simulink model "active_stereo_ibvs"  (R2025b)
settings: Solver=FixedStepDiscrete  StartTime=0.0  StopTime=Tstop  FixedStep=Ts  RelTol=1e-3
values from neighbouring files (symbols this model uses):
  Ts = cfg.Ts;'    [build_arm_stereo_ibvs_ekf_v1.m]
undefined symbols (not defined in the file or in its folder): adaptEnable, cam, dhatn0, DiscIntNeverNeededParam, experimentMode, featureScale, feedforwardEnable, gammaRho, lambda, mu, q0, qmax, qmin, rateScale, rho0, rhomax, rhomin, sd, sdDot, sigmaRho, target0, trajParam
settings Model: Creator=ASUS  LastModifiedBy=ASUS

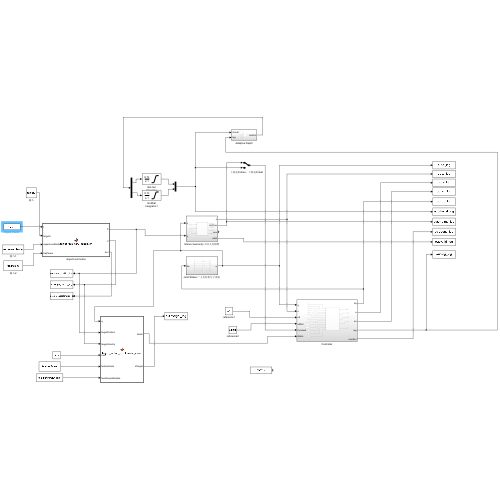
[thumbnail: Simulink's stored preview of the top-level diagram]
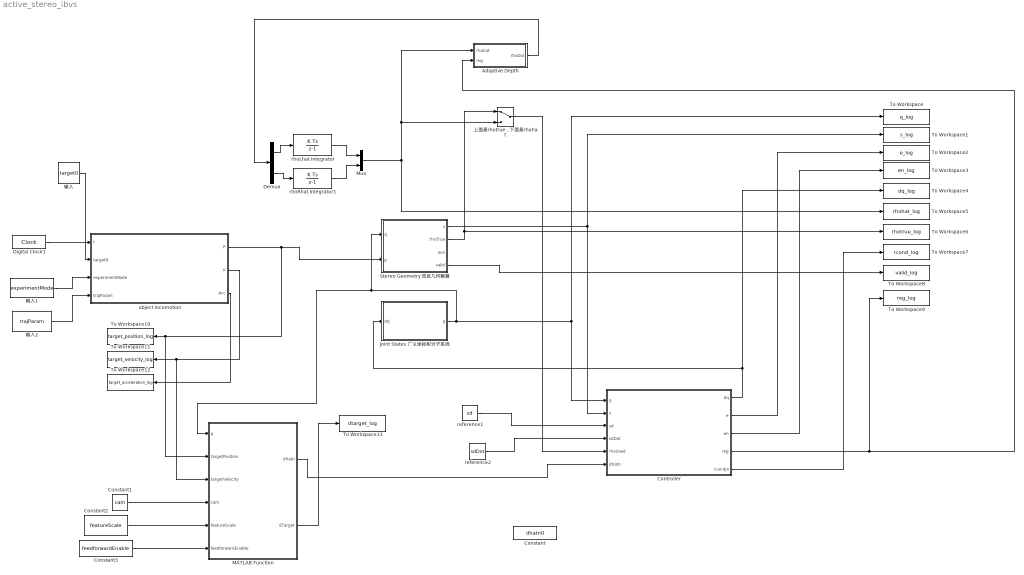
== system active_stereo_ibvs ==
  Adaptive Depth : Subsystem
  Constant : Constant  Value=dhatn0
  Constant1 : Constant  Value=cam
  Constant2 : Constant  Value=featureScale
  Constant3 : Constant  Value=feedforwardEnable
  Controller : Subsystem
  Demux : Demux  Outputs=2
  Digital Clock1 : DigitalClock  SampleTime=Ts
  Joint States 广义坐标积分子系统 : Subsystem
  MATLAB Function : MATLAB Function  TreatAsAtomicUnit=on
  Mux : Mux  Inputs=2
  Stereo Geometry 双目几何解算 : Subsystem
  To Workspace : ToWorkspace  VariableName=q_log  SaveFormat=Timeseries  SampleTime=-1
  To Workspace1 : ToWorkspace  VariableName=s_log  SaveFormat=Timeseries  SampleTime=-1
  To Workspace10 : ToWorkspace  VariableName=target_position_log  SaveFormat=Timeseries  SampleTime=-1
  To Workspace11 : ToWorkspace  VariableName=target_velocity_log  SaveFormat=Timeseries  SampleTime=-1
  To Workspace12 : ToWorkspace  VariableName=target_acceleration_log  SaveFormat=Timeseries  SampleTime=-1
  To Workspace13 : ToWorkspace  VariableName=dtarget_log  SaveFormat=Timeseries  SampleTime=-1
  To Workspace2 : ToWorkspace  VariableName=e_log  SaveFormat=Timeseries  SampleTime=-1
  To Workspace3 : ToWorkspace  VariableName=en_log  SaveFormat=Timeseries  SampleTime=-1
  To Workspace4 : ToWorkspace  VariableName=dq_log  SaveFormat=Timeseries  SampleTime=-1
  To Workspace5 : ToWorkspace  VariableName=rhohat_log  SaveFormat=Timeseries  SampleTime=-1
  To Workspace6 : ToWorkspace  VariableName=rhotrue_log  SaveFormat=Timeseries  SampleTime=-1
  To Workspace7 : ToWorkspace  VariableName=rcond_log  SaveFormat=Timeseries  SampleTime=-1
  To Workspace8 : ToWorkspace  VariableName=valid_log  SaveFormat=Timeseries  SampleTime=-1
  To Workspace9 : ToWorkspace  VariableName=reg_log  SaveFormat=Timeseries  SampleTime=-1
  object locomotion : MATLAB Function  TreatAsAtomicUnit=on
  reference1 : Constant  Value=sd
  reference2 : Constant  Value=sdDot
  rhoLhat Integrator : DiscreteIntegrator  InitialCondition=rho0(1)  SampleTime=Ts  LimitOutput=on  UpperSaturationLimit=rhomax(1)  LowerSaturationLimit=rhomin(1)  ICPrevOutput=DiscIntNeverNeededParam  ICPrevScaledInput=DiscIntNeverNeededParam
  rhoRhat Integrator1 : DiscreteIntegrator  InitialCondition=rho0(2)  SampleTime=Ts  LimitOutput=on  UpperSaturationLimit=rhomax(2)  LowerSaturationLimit=rhomin(2)  ICPrevOutput=DiscIntNeverNeededParam  ICPrevScaledInput=DiscIntNeverNeededParam
  上面是rhotrue，下面是rhohat : ManualSwitch
  输入 : Constant  Value=target0
  输入1 : Constant  Value=experimentMode
  输入2 : Constant  Value=trajParam
  wires:
  rhoLhat Integrator/1 -> Mux/1
  rhoRhat Integrator1/1 -> Mux/2
  Mux/1 -> Adaptive Depth/1(rhohat), 上面是rhotrue，下面是rhohat/2, To Workspace5/1
  Controller/1(dq) -> To Workspace4/1, Joint States 广义坐标积分子系统/1(dq)
  Stereo Geometry 双目几何解算/2(rhoTrue) -> To Workspace6/1, 上面是rhotrue，下面是rhohat/1
  上面是rhotrue，下面是rhohat/1 -> Controller/5(rhoUsed)
  Joint States 广义坐标积分子系统/1(q) -> MATLAB Function/1(q), Stereo Geometry 双目几何解算/1(q), Controller/1(q), To Workspace/1
  Stereo Geometry 双目几何解算/1(s) -> Controller/2(s), To Workspace1/1
  Controller/2(e) -> To Workspace2/1
  Controller/3(en) -> To Workspace3/1
  Controller/5(rcondJn) -> To Workspace7/1
  Stereo Geometry 双目几何解算/4(valid) -> To Workspace8/1
  Demux/1 -> rhoLhat Integrator/1
  Demux/2 -> rhoRhat Integrator1/1
  Adaptive Depth/1(rhoDot) -> Demux/1
  Controller/4(reg) -> To Workspace9/1, Adaptive Depth/2(reg)
  reference1/1 -> Controller/3(sd)
  reference2/1 -> Controller/4(sdDot)
  Digital Clock1/1 -> object locomotion/1(t)
  输入/1 -> object locomotion/2(target0)
  输入1/1 -> object locomotion/3(experimentMode)
  输入2/1 -> object locomotion/4(trajParam)
  object locomotion/1(P) -> MATLAB Function/2(targetPosition), To Workspace10/1, Stereo Geometry 双目几何解算/2(p)
  object locomotion/2(V) -> MATLAB Function/3(targetVelocity), To Workspace11/1
  object locomotion/3(Acc) -> To Workspace12/1
  Constant1/1 -> MATLAB Function/4(cam)
  Constant2/1 -> MATLAB Function/5(featureScale)
  Constant3/1 -> MATLAB Function/6(feedforwardEnable)
  MATLAB Function/2(dTarget) -> To Workspace13/1
  MATLAB Function/1(dhatn) -> Controller/6(dhatn)

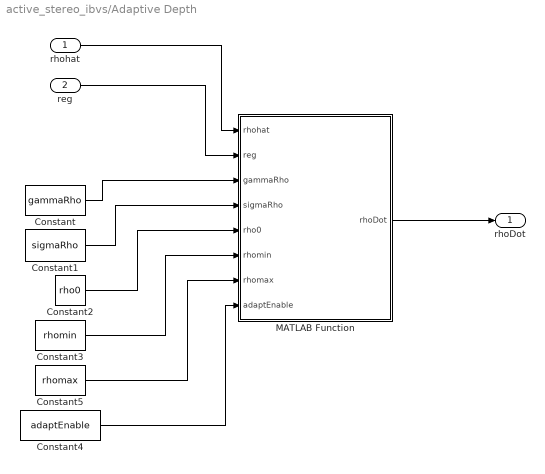
== system active_stereo_ibvs/Adaptive Depth ==
  rhohat : Inport
  reg : Inport  Port=2
  Constant : Constant  Value=gammaRho
  Constant1 : Constant  Value=sigmaRho
  Constant2 : Constant  Value=rho0
  Constant3 : Constant  Value=rhomin
  Constant4 : Constant  Value=adaptEnable
  Constant5 : Constant  Value=rhomax
  MATLAB Function : MATLAB Function  TreatAsAtomicUnit=on
  rhoDot : Outport
  wires:
  rhohat/1 -> MATLAB Function/1(rhohat)
  reg/1 -> MATLAB Function/2(reg)
  MATLAB Function/1(rhoDot) -> rhoDot/1
  Constant/1 -> MATLAB Function/3(gammaRho)
  Constant1/1 -> MATLAB Function/4(sigmaRho)
  Constant2/1 -> MATLAB Function/5(rho0)
  Constant3/1 -> MATLAB Function/6(rhomin)
  Constant5/1 -> MATLAB Function/7(rhomax)
  Constant4/1 -> MATLAB Function/8(adaptEnable)

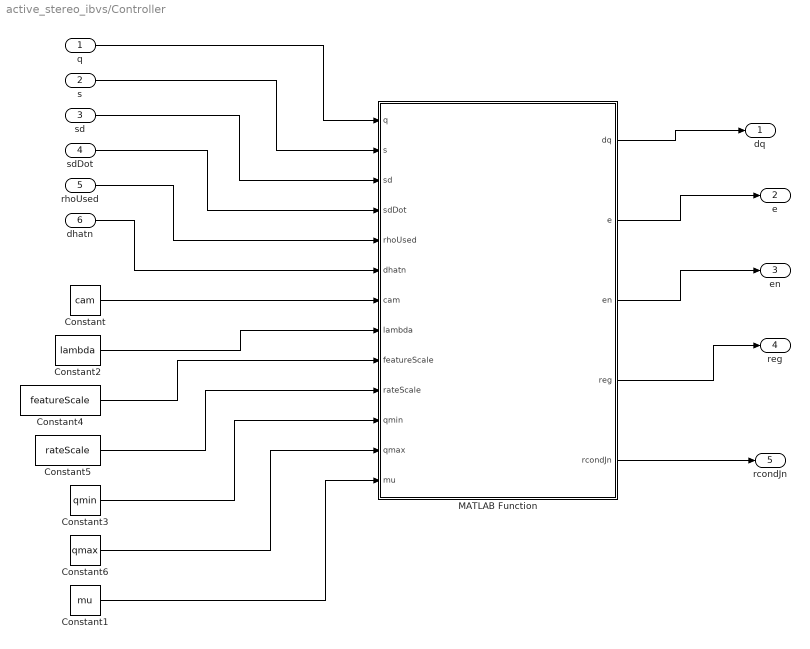
== system active_stereo_ibvs/Controller ==
  q : Inport
  s : Inport  Port=2
  sd : Inport  Port=3
  sdDot : Inport  Port=4
  rhoUsed : Inport  Port=5
  dhatn : Inport  Port=6
  Constant : Constant  Value=cam
  Constant1 : Constant  Value=mu
  Constant2 : Constant  Value=lambda
  Constant3 : Constant  Value=qmin  VectorParams1D=off
  Constant4 : Constant  Value=featureScale
  Constant5 : Constant  Value=rateScale
  Constant6 : Constant  Value=qmax
  MATLAB Function : MATLAB Function  TreatAsAtomicUnit=on
  dq : Outport
  e : Outport  Port=2
  en : Outport  Port=3
  reg : Outport  Port=4
  rcondJn : Outport  Port=5
  wires:
  q/1 -> MATLAB Function/1(q)
  s/1 -> MATLAB Function/2(s)
  sd/1 -> MATLAB Function/3(sd)
  sdDot/1 -> MATLAB Function/4(sdDot)
  rhoUsed/1 -> MATLAB Function/5(rhoUsed)
  dhatn/1 -> MATLAB Function/6(dhatn)
  Constant/1 -> MATLAB Function/7(cam)
  Constant2/1 -> MATLAB Function/8(lambda)
  Constant4/1 -> MATLAB Function/9(featureScale)
  Constant5/1 -> MATLAB Function/10(rateScale)
  Constant3/1 -> MATLAB Function/11(qmin)
  Constant6/1 -> MATLAB Function/12(qmax)
  Constant1/1 -> MATLAB Function/13(mu)
  MATLAB Function/1(dq) -> dq/1
  MATLAB Function/2(e) -> e/1
  MATLAB Function/3(en) -> en/1
  MATLAB Function/4(reg) -> reg/1
  MATLAB Function/5(rcondJn) -> rcondJn/1

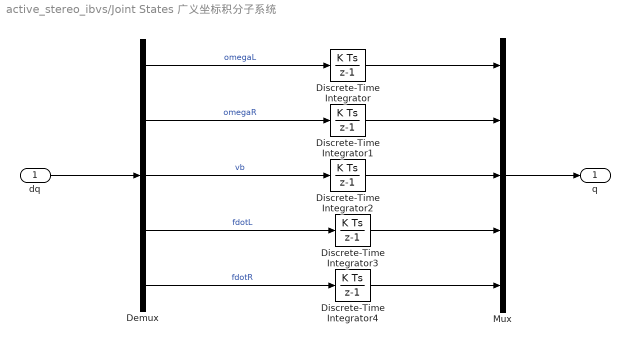
== system active_stereo_ibvs/Joint States 广义坐标积分子系统 ==
  dq : Inport
  Demux : Demux  Outputs=5
  Discrete-Time Integrator : DiscreteIntegrator  InitialCondition=q0(1)  SampleTime=Ts  LimitOutput=on  UpperSaturationLimit=qmax(1)  LowerSaturationLimit=qmin(1)  ICPrevOutput=DiscIntNeverNeededParam  ICPrevScaledInput=DiscIntNeverNeededParam
  Discrete-Time Integrator1 : DiscreteIntegrator  InitialCondition=q0(2)  SampleTime=Ts  LimitOutput=on  UpperSaturationLimit=qmax(2)  LowerSaturationLimit=qmin(2)  ICPrevOutput=DiscIntNeverNeededParam  ICPrevScaledInput=DiscIntNeverNeededParam
  Discrete-Time Integrator2 : DiscreteIntegrator  InitialCondition=q0(3)  SampleTime=Ts  LimitOutput=on  UpperSaturationLimit=qmax(3)  LowerSaturationLimit=qmin(3)  ICPrevOutput=DiscIntNeverNeededParam  ICPrevScaledInput=DiscIntNeverNeededParam
  Discrete-Time Integrator3 : DiscreteIntegrator  InitialCondition=q0(4)  SampleTime=Ts  LimitOutput=on  UpperSaturationLimit=qmax(4)  LowerSaturationLimit=qmin(4)  ICPrevOutput=DiscIntNeverNeededParam  ICPrevScaledInput=DiscIntNeverNeededParam
  Discrete-Time Integrator4 : DiscreteIntegrator  InitialCondition=q0(5)  SampleTime=Ts  LimitOutput=on  UpperSaturationLimit=qmax(5)  LowerSaturationLimit=qmin(5)  ICPrevOutput=DiscIntNeverNeededParam  ICPrevScaledInput=DiscIntNeverNeededParam
  Mux : Mux  Inputs=5
  q : Outport
  wires:
  Demux/4 -> Discrete-Time Integrator3/1  "fdotL"
  Demux/3 -> Discrete-Time Integrator2/1  "vb"
  Demux/5 -> Discrete-Time Integrator4/1  "fdotR"
  Discrete-Time Integrator4/1 -> Mux/5
  Discrete-Time Integrator1/1 -> Mux/2
  Discrete-Time Integrator/1 -> Mux/1
  Discrete-Time Integrator2/1 -> Mux/3
  Discrete-Time Integrator3/1 -> Mux/4
  Demux/2 -> Discrete-Time Integrator1/1  "omegaR"
  Demux/1 -> Discrete-Time Integrator/1  "omegaL"
  dq/1 -> Demux/1
  Mux/1 -> q/1

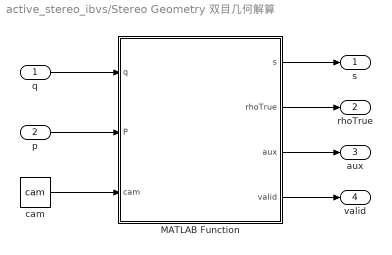
== system active_stereo_ibvs/Stereo Geometry 双目几何解算 ==
  q : Inport
  p : Inport  Port=2
  MATLAB Function : MATLAB Function  TreatAsAtomicUnit=on
  cam : Constant  Value=cam
  s : Outport
  rhoTrue : Outport  Port=2
  aux : Outport  Port=3
  valid : Outport  Port=4
  wires:
  q/1 -> MATLAB Function/1(q)
  p/1 -> MATLAB Function/2(P)
  cam/1 -> MATLAB Function/3(cam)
  MATLAB Function/1(s) -> s/1
  MATLAB Function/2(rhoTrue) -> rhoTrue/1
  MATLAB Function/3(aux) -> aux/1
  MATLAB Function/4(valid) -> valid/1

== matlab function active_stereo_ibvs/Controller/MATLAB Function ==
  data: q input; dq output size=[5 1]; s input; sd input; sdDot input; rhoUsed input; dhatn input; cam input; lambda input; featureScale input; rateScale input; qmin input; qmax input; mu input; e output; en output; reg output; rcondJn output
function [dq, e, en, reg, rcondJn] = controller5( ...
    q, s, sd, sdDot, rhoUsed, dhatn, ...
    cam, lambda, featureScale, rateScale, qmin, qmax, mu)
%#codegen
%
% q  = [alphaL; alphaR; b; fL; fR]
% s  = [uL; aL; uR; aR; b]
% dq = [omegaL; omegaR; vb; fdotL; fdotR]

%% 固定输出尺寸
dq = zeros(5,1);
e = zeros(5,1);
en = zeros(5,1);
reg = zeros(2,1);
rcondJn = 0.0;

%% 固定中间变量尺寸
W = zeros(5,5);
Du = zeros(5,5);
Jhat = zeros(5,5);
Jn = zeros(5,5);
G = zeros(5,5);
rhs = zeros(5,1);
z = zeros(5,1);

JL = zeros(5,5);
JR = zeros(5,5);
phiL = zeros(5,1);
phiR = zeros(5,1);

%% 读取状态
alphaL = q(1);
alphaR = q(2);

fL = q(4);
fR = q(5);

uL = s(1);
aL = s(2);
uR = s(3);
aR = s(4);

cxL = cam(1);
cxR = cam(2);

rhoL = rhoUsed(1);
rhoR = rhoUsed(2);

sigmaL = -1.0;
sigmaR =  1.0;

%% 归一化图像坐标
fLsafe = max(fL,1.0);
fRsafe = max(fR,1.0);

xL = (uL-cxL)/fLsafe;
xR = (uR-cxR)/fRsafe;

%% 旋转雅可比
AL = -fL*(1.0+xL*xL);
AR = -fR*(1.0+xR*xR);

CL = -aL*xL;
CR = -aR*xR;

%% 基线雅可比
BbarL = sigmaL*fL/2.0 * ...
    (-cos(alphaL)+xL*sin(alphaL));

BbarR = sigmaR*fR/2.0 * ...
    (-cos(alphaR)+xR*sin(alphaR));

DbarL = sigmaL*aL/2.0*sin(alphaL);
DbarR = sigmaR*aR/2.0*sin(alphaR);

%% 构造估计雅可比
Jhat(1,1) = AL;
Jhat(1,3) = rhoL*BbarL;
Jhat(1,4) = xL;

Jhat(2,1) = CL;
Jhat(2,3) = rhoL*DbarL;
Jhat(2,4) = aL/fLsafe;

Jhat(3,2) = AR;
Jhat(3,3) = rhoR*BbarR;
Jhat(3,5) = xR;

Jhat(4,2) = CR;
Jhat(4,3) = rhoR*DbarR;
Jhat(4,5) = aR/fRsafe;

Jhat(5,3) = 1.0;

%% 特征误差：实际减期望
for k = 1:5
    e(k) = s(k)-sd(k);
end

%% 归一化矩阵
for k = 1:5
    W(k,k) = 1.0/featureScale(k);
    Du(k,k) = rateScale(k);
end

en = W*e;
Jn = W*Jhat*Du;

%% 期望归一化特征速度
for k = 1:5
    rhs(k) = sdDot(k)/featureScale(k) ...
           - lambda(k)*en(k) ...
           - dhatn(k);
end

%% 阻尼最小二乘
G = Jn*Jn' + mu*mu*eye(5);

z = Jn'*(G\rhs);

%% 归一化输入限幅
for k = 1:5
    if z(k) > 1.0
        z(k) = 1.0;
    elseif z(k) < -1.0
        z(k) = -1.0;
    end
end

%% 转换成实际控制输入
for k = 1:5
    dq(k) = rateScale(k)*z(k);
end

%% 状态边界保护
epsq = 1e-8;

for k = 1:5
    if q(k) <= qmin(k)+epsq && dq(k) < 0.0
        dq(k) = 0.0;
    end

    if q(k) >= qmax(k)-epsq && dq(k) > 0.0
        dq(k) = 0.0;
    end
end

%% 逆深度自适应回归矩阵
JL(1,3) = BbarL;
JL(2,3) = DbarL;

JR(3,3) = BbarR;
JR(4,3) = DbarR;

phiL = W*(JL*dq);
phiR = W*(JR*dq);

reg(1) = phiL'*en;
reg(2) = phiR'*en;

%% 雅可比条件数监测
rcondJn = rcond(Jn);

end

== matlab function active_stereo_ibvs/Stereo Geometry 双目几何解算/MATLAB Function ==
  data: q input; s output; P input; cam input; rhoTrue output; aux output; valid output
function [s, rhoTrue, aux, valid] = stereo_geometry(q, P, cam)
%#codegen
%
% q = [alphaL; alphaR; b; fL; fR]
% P = [XB; YB; ZB]
% cam = [cxL; cxR; kL; kR; imageWidth]
%
% s = [uL; aL; uR; aR; b]
% rhoTrue = [rhoL; rhoR]
% aux = [xL; xR; ZL; ZR]

alphaL = q(1);
alphaR = q(2);
b      = q(3);
fL     = q(4);
fR     = q(5);

cxL = cam(1);
cxR = cam(2);
kL  = cam(3);
kR  = cam(4);
imageWidth = cam(5);

sigmaL = -1.0;
sigmaR =  1.0;

%% 左相机坐标变换
% 左相机中心 C_L = [-b/2;0;0]
dxL = P(1) - sigmaL*b/2;
dyL = P(2);
dzL = P(3);

cL = cos(alphaL);
sL = sin(alphaL);

% P_L = R_y(alphaL)' * (P-C_L)
XL = cL*dxL - sL*dzL;
YL = dyL;
ZL = sL*dxL + cL*dzL;

%% 右相机坐标变换
dxR = P(1) - sigmaR*b/2;
dyR = P(2);
dzR = P(3);

cR = cos(alphaR);
sR = sin(alphaR);

XR = cR*dxR - sR*dzR;
YR = dyR;
ZR = sR*dxR + cR*dzR;

%% 防止除零
Zmin = 0.05;

valid = 1.0;

if ZL <= Zmin || ZR <= Zmin
    valid = 0.0;
end

ZLsafe = max(ZL, Zmin);
ZRsafe = max(ZR, Zmin);

%% 归一化坐标
xL = XL/ZLsafe;
xR = XR/ZRsafe;

%% 图像特征
uL = cxL + fL*xL;
uR = cxR + fR*xR;

aL = kL*fL/ZLsafe;
aR = kR*fR/ZRsafe;

if uL < 0 || uL > imageWidth || ...
   uR < 0 || uR > imageWidth
    valid = 0.0;
end

%% 输出
s = zeros(5,1);
s(1) = uL;
s(2) = aL;
s(3) = uR;
s(4) = aR;
s(5) = b;

rhoTrue = zeros(2,1);
rhoTrue(1) = 1/ZLsafe;
rhoTrue(2) = 1/ZRsafe;

aux = zeros(4,1);
aux(1) = xL;
aux(2) = xR;
aux(3) = ZL;
aux(4) = ZR;
end

== matlab function active_stereo_ibvs/Adaptive Depth/MATLAB Function ==
  data: rhohat input; rhoDot output; reg input; gammaRho input; sigmaRho input; rho0 input; rhomin input; rhomax input; adaptEnable input
function rhoDot = adaptive_depth( ...
    rhohat, reg, gammaRho, sigmaRho, ...
    rho0, rhomin, rhomax, adaptEnable)
%#codegen

rhoDot = zeros(2,1);

if adaptEnable < 0.5
    return;
end

for k = 1:2
    rhoDot(k) = gammaRho(k)*reg(k) ...
              - sigmaRho(k)*(rhohat(k)-rho0(k));

    % 投影保护
    if rhohat(k) <= rhomin(k) && rhoDot(k) < 0
        rhoDot(k) = 0;
    end

    if rhohat(k) >= rhomax(k) && rhoDot(k) > 0
        rhoDot(k) = 0;
    end
end
end

== matlab function active_stereo_ibvs/MATLAB Function ==
  data: q input double; dhatn output double; targetPosition input double; targetVelocity input double; cam input double; featureScale input double; feedforwardEnable input double; dTarget output double
function [dhatn, dTarget] = target_motion_feedforward_exact( ...
    q, targetPosition, targetVelocity, ...
    cam, featureScale, feedforwardEnable)
%#codegen
%
% 快速移动目标的理想速度前馈
%
% 本函数直接按照 Stereo Geometry 中的相机几何重新计算：
% 1. 目标在左右相机坐标系中的位置；
% 2. 左右相机的真实逆深度；
% 3. 目标速度在左右相机坐标系中的分量；
% 4. 目标运动造成的图像特征变化率。
%
% 这样可以避免 s、rhoTrue 等外部信号接错或不同步。
%
% 输入：
% q =
%   [alphaL;
%    alphaR;
%    b;
%    fL;
%    fR]
%
% targetPosition =
%   [X;
%    Y;
%    Z]
%
% targetVelocity =
%   [VX;
%    VY;
%    VZ]
%
% cam =
%   [cxL;
%    cxR;
%    kL;
%    kR;
%    imageWidth]
%
% featureScale：
%   五个视觉特征的归一化尺度
%
% feedforwardEnable：
%   1：开启理想目标速度前馈
%   0：关闭目标速度前馈
%
% 输出：
% dTarget：
%   未归一化的目标运动特征速度
%
% dhatn：
%   归一化目标运动特征速度，
%   直接连接 Controller 的 dhatn 输入

%% =========================================================
% 1. 输出初始化
% ==========================================================

dhatn = zeros(5,1);
dTarget = zeros(5,1);

%% =========================================================
% 2. 前馈关闭
% ==========================================================

if feedforwardEnable < 0.5
    return;
end

%% =========================================================
% 3. 提取系统状态
% ==========================================================

alphaL = q(1);
alphaR = q(2);

b = q(3);

fL = q(4);
fR = q(5);

%% =========================================================
% 4. 提取目标位置和速度
% ==========================================================

X = targetPosition(1);
Y = targetPosition(2);
Z = targetPosition(3);

VX = targetVelocity(1);
VY = targetVelocity(2);
VZ = targetVelocity(3);

%% =========================================================
% 5. 提取相机参数
% ==========================================================

cxL = cam(1);
cxR = cam(2);

kL = cam(3);
kR = cam(4);

%% =========================================================
% 6. 左右相机位置符号
%
% 左相机中心：[-b/2, 0, 0]
% 右相机中心：[+b/2, 0, 0]
% ==========================================================

sigmaL = -1.0;
sigmaR = 1.0;

%% =========================================================
% 7. 数值安全参数
% ==========================================================

Zminimum = 0.05;

fLsafe = max(abs(fL), 1.0);
fRsafe = max(abs(fR), 1.0);

%% =========================================================
% 8. 目标相对于左相机光心的位置
% ==========================================================

dxL = X - sigmaL*b/2.0;
dyL = Y;
dzL = Z;

cosL = cos(alphaL);
sinL = sin(alphaL);

XL = cosL*dxL - sinL*dzL;
YL = dyL;
ZL = sinL*dxL + cosL*dzL;

ZLsafe = max(ZL, Zminimum);

rhoL = 1.0/ZLsafe;
xL = XL/ZLsafe;

%% =========================================================
% 9. 目标相对于右相机光心的位置
% ==========================================================

dxR = X - sigmaR*b/2.0;
dyR = Y;
dzR = Z;

cosR = cos(alphaR);
sinR = sin(alphaR);

XR = cosR*dxR - sinR*dzR;
YR = dyR;
ZR = sinR*dxR + cosR*dzR;

ZRsafe = max(ZR, Zminimum);

rhoR = 1.0/ZRsafe;
xR = XR/ZRsafe;

%% =========================================================
% 10. 当前图像特征
%
% 虽然水平坐标本身未直接用于输出，
% 但在这里完整计算，便于保证与 Geometry 一致。
% ==========================================================

uL = cxL + fL*xL;
uR = cxR + fR*xR;

aL = kL*fL/ZLsafe;
aR = kR*fR/ZRsafe;

% 防止代码生成阶段将变量视为未使用
uL = uL + 0.0;
uR = uR + 0.0;
YL = YL + 0.0;
YR = YR + 0.0;
VY = VY + 0.0;

%% =========================================================
% 11. 世界坐标系速度转换到左相机坐标系
%
% 与 Stereo Geometry 中的位置变换严格一致：
%
% XL = cos(alphaL)*dxL - sin(alphaL)*dzL
% ZL = sin(alphaL)*dxL + cos(alphaL)*dzL
% ==========================================================

VXL = cosL*VX - sinL*VZ;
VYL = VY;
VZL = sinL*VX + cosL*VZ;

%% =========================================================
% 12. 世界坐标系速度转换到右相机坐标系
% ==========================================================

VXR = cosR*VX - sinR*VZ;
VYR = VY;
VZR = sinR*VX + cosR*VZ;

% 当前模型不使用竖直图像坐标，但保留变量
VYL = VYL + 0.0;
VYR = VYR + 0.0;

%% =========================================================
% 13. 左相机目标运动特征速度
%
% u = cx + f*X/Z
%
% du_target =
%     f/Z * (VX_camera - x*VZ_camera)
%
% a = k*f/Z
%
% da_target =
%     -a/Z * VZ_camera
% ==========================================================

duTargetL = ...
    fL*rhoL*(VXL-xL*VZL);

daTargetL = ...
    -aL*rhoL*VZL;

%% =========================================================
% 14. 右相机目标运动特征速度
% ==========================================================

duTargetR = ...
    fR*rhoR*(VXR-xR*VZR);

daTargetR = ...
    -aR*rhoR*VZR;

%% =========================================================
% 15. 构造目标运动特征速度
%
% 第五个特征为机械基线。
% 目标运动不会直接改变机械基线，所以第五项为0。
% ==========================================================

dTarget(1) = duTargetL;
dTarget(2) = daTargetL;
dTarget(3) = duTargetR;
dTarget(4) = daTargetR;
dTarget(5) = 0.0;

%% =========================================================
% 16. 归一化
%
% Controller 内部使用：
%
% rhs =
%   W*sdDot
%   - Lambda*en
%   - dhatn
%
% 因此这里需要输出：
%
% dhatn = W*dTarget
% ==========================================================

for index = 1:5

    scaleSafe = max( ...
        abs(featureScale(index)), ...
        1.0e-9);

    dhatn(index) = ...
        dTarget(index)/scaleSafe;

end

end

== matlab function active_stereo_ibvs/object locomotion ==
  data: t input double; P output double; target0 input double; V output double; experimentMode input double; trajParam input double; Acc output double
function [P, V, Acc] = target_trajectory_generator( ...
    t, target0, experimentMode, trajParam)
%#codegen
%
% 动态目标轨迹发生器
%
% 输入：
% t               当前仿真时间，标量
% target0         目标中心位置 [X0;Y0;Z0]
% experimentMode  实验编号：7、8、9或10
% trajParam       轨迹参数：
%                 [Ax; wx; Az; wz; phaseZ; Ttriangle]
%
% 输出：
% P     目标位置 [X;Y;Z]
% V     目标速度 [Vx;Vy;Vz]
% Acc   目标加速度 [Ax;Ay;Az]

P = zeros(3,1);
V = zeros(3,1);
Acc = zeros(3,1);

X0 = target0(1);
Y0 = target0(2);
Z0 = target0(3);

horizontalAmplitude = trajParam(1);
horizontalOmega = trajParam(2);

depthAmplitude = trajParam(3);
depthOmega = trajParam(4);
depthPhase = trajParam(5);

trianglePeriod = trajParam(6);

% 默认目标保持静止
P(1) = X0;
P(2) = Y0;
P(3) = Z0;

mode = int32(experimentMode);

switch mode

    case 7
        % ====================================================
        % 实验七：目标横向正弦运动
        % X(t) = X0 + Ax*sin(wx*t)
        % ====================================================

        P(1) = X0 + ...
            horizontalAmplitude * sin(horizontalOmega*t);

        V(1) = horizontalAmplitude * horizontalOmega * ...
            cos(horizontalOmega*t);

        Acc(1) = -horizontalAmplitude * ...
            horizontalOmega^2 * sin(horizontalOmega*t);

    case 8
        % ====================================================
        % 实验八：目标前后深度正弦运动
        % Z(t) = Z0 + Az*sin(wz*t)
        % ====================================================

        P(3) = Z0 + ...
            depthAmplitude * sin(depthOmega*t + depthPhase);

        V(3) = depthAmplitude * depthOmega * ...
            cos(depthOmega*t + depthPhase);

        Acc(3) = -depthAmplitude * depthOmega^2 * ...
            sin(depthOmega*t + depthPhase);

    case 9
        % ====================================================
        % 实验九：横向与前后复合运动
        % ====================================================

        P(1) = X0 + ...
            horizontalAmplitude * sin(horizontalOmega*t);

        V(1) = horizontalAmplitude * horizontalOmega * ...
            cos(horizontalOmega*t);

        Acc(1) = -horizontalAmplitude * ...
            horizontalOmega^2 * sin(horizontalOmega*t);

        P(3) = Z0 + ...
            depthAmplitude * sin(depthOmega*t + depthPhase);

        V(3) = depthAmplitude * depthOmega * ...
            cos(depthOmega*t + depthPhase);

        Acc(3) = -depthAmplitude * depthOmega^2 * ...
            sin(depthOmega*t + depthPhase);

    case 10
        % ====================================================
        % 实验十：横向三角波运动
        %
        % 目标以恒定速度左右往返，在端点突然反向。
        % 这是压力测试，端点处速度会瞬间反向。
        % ====================================================

        safePeriod = max(trianglePeriod, 0.1);

        % 加入1/4周期相位，使t=0时目标位于X0
        tau = mod(t + 0.25*safePeriod, safePeriod);

        halfPeriod = 0.5*safePeriod;

        % 三角波最大速度
        triangleSpeed = ...
            4.0*horizontalAmplitude/safePeriod;

        if tau < halfPeriod

            P(1) = X0 - horizontalAmplitude + ...
                triangleSpeed*tau;

            V(1) = triangleSpeed;

        else

            P(1) = X0 + horizontalAmplitude - ...
                triangleSpeed*(tau-halfPeriod);

            V(1) = -triangleSpeed;

        end

        % 三角波端点加速度理论上不连续。
        % 这里只记录非端点区间为0。
        Acc(1) = 0.0;

    otherwise
        % 其他模式保持静止目标
end

end
